simulink library "Storage_Type_5"  (R2018b)
settings: Solver=ode45  StartTime=0.0  StopTime=10.0  RelTol=1e-3  EnableMultiTasking=on
undefined symbols (not defined in the file): path_carnot
libraries: carnot x12
settings Model: Creator=bernd.hafner  LastModifiedBy=drhf
settings DataIOCC: LimitDataPoints=on  SaveFormat=Array  SignalLoggingSaveFormat=ModelDataLogs
settings OptimizationCC: ExpressionDepthLimit=2147483647  LifeSpan=inf
settings DebuggingCC: UnderspecifiedInitializationDetection=Classic  MergeDetectMultiDrivingBlocksExec=none  SolverPrmCheckMsg=warning  FcnCallInpInsideContextMsg=warning  StateNameClashWarn=warning  SFUnexpectedBacktrackingDiag=warning  SFNoUnconditionalDefaultTransitionDiag=warning  SFExecutionAtInitializationDiag=none
settings HardwareCC: ProdBitPerPointer=32  ProdBitPerSizeT=32  ProdBitPerPtrDiffT=32  ProdLargestAtomicFloat=None  ProdIntDivRoundTo=Undefined  ProdEndianess=Unspecified  ProdWordSize=32  ProdHWDeviceType=32-bit Generic
settings ModelReferenceCC: PropagateSignalLabelsOutOfModel=off
settings SFSimCC: SimUseLocalCustomCode=off
settings RTWCC: RTWUseLocalCustomCode=off
settings CodeAppCC: StateflowObjectComments=on
settings GRTTargetCC: TargetLangStandard=C89/C90 (ANSI)  CombineOutputUpdateFcns=off  GRTInterface=on
settings ConfigComp: CovMetricSettings=dw  CovHtmlReporting=on  CovSaveCumulativeToWorkspaceVar=on  CovSaveSingleToWorkspaceVar=on  CovExternalEMLEnable=off

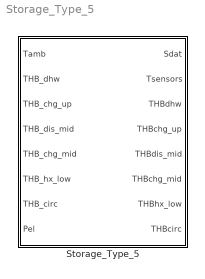
== system Storage_Type_5 ==
  Storage_Type_5 : Subsystem  mask(Combi-storage for hot water production and heating){t0=[10:5:55], hgt=1.7623, stgtype=5, tini=[10 12.3684210526316 14.7368421052632 17.1052631578947 19.4736842105263 21.8421052631579 24.2105263157895 26.5789473684211 28.9473684210526 31.3157894736842 33.6842105263158 36.0526315789474 38.4210526315789 40.7894736842105 43.1578947368421 45.5263157894737 47.8947368421053 50.2631578947368 52.6315789473684 55], mpts=[1 3 5 7 9 11 13 15 17 19], PathName=fullfile(path_carnot('libsl'), 'Storage', 'Thermal', 'Storage_Type_5', 'parameter_set'), FileName='StorageType5_800_L.mat', userPath=off, userParam=off, uwall=1, ubot=1, utop=1, axcond=1, volume=1, dia=0.85, standing=standing cylinder, nodes=20, mpoints=10, Tsensor=[0.2 0.5 0.7], pipe3inlet=1, pipe3outlet=0.6, pipe3dia=0.05, pipe1inlet=0.55, pipe1outlet=0.45, pipe1dia=0.05, hx1inlet=0.4, hx1outlet=0, hx1dia=0.03, hx1uac=200, hx1uam=0.15, hx1uat=0.6, hx1_uat2=0, hx1dplin=20, hx1dpqua=20, pipe2inlet=0.45, pipe2outlet=0.55, pipe2dia=0.05, hx2inlet=0, hx2outlet=1, hx2dia=0.025, hx2uac=450, hx2uam=0.4, hx2uat=0.8, hx2_uat2=0, hx2dplin=200, hx2dpqua=200, hx3inlet=0.9, hx3outlet=1, hx3dia=0.01, hx3uac=100, hx3uam=0, hx3uat=0, hx3_uat2=0, hx3dplin=10, hx3dpqua=10, heater1start=0.6, heater1end=0.65}
      mask prompts: t0 "Initial temperature (vector or scalar) in °C"; hgt "Height of storage in m"; stgtype "Storage Type (0..5)"; tini "Start temperatures of nodes in °C"; mpts "Index to measured nodes"; PathName "Path"; FileName "Parameter set"; userPath "Edit path and name of parameter set"; userParam "User defined parameters"; uwall "Heat transfer coefficient to ambient [W/m²K]"; ubot "Heat transfer coefficient to ambient bottom [W/m²K]"; utop "Heat transfer coefficient to ambient top [W/m²K]"; axcond "Effective thermal conductivity [W/m/K]"; volume "Volume [m³]"; dia "Diameter [m]"; standing "Position"; nodes "Number of nodes"; mpoints "Number of node temperatures (for display)"; Tsensor "Temperature sensor position (0..1, 0 = bottom, 1 = top)"; pipe3inlet "relative height of inlet, range from 0 (= bottom) to 1 (= top)"; pipe3outlet "relative height of outlet, range from 0 (= bottom) to 1 (= top)"; pipe3dia "Diameter of pipe in m"; pipe1inlet "relative height of inlet, range from 0 (= bottom) to 1 (= top)"; pipe1outlet "relative height of outlet, range from 0 (= bottom) to 1 (= top)"; pipe1dia "Diameter of pipe in m"; hx1inlet "relative height of inlet"; hx1outlet "relative height of outlet"; hx1dia "Diameter of HX pipe [m]"; hx1uac "uac: heat transfer coefficient [W/K /(kg/s) /(°C)]"; hx1uam "uam: massflow dependent heat transfer [-]"; hx1uat "uat: temperature dependent heat transfer [-]"; hx1_uat2 "uat2: temperature difference dependent heat transfer [-]"; hx1dplin "pressure drop linear in mdot [Pa*s/kg]"; hx1dpqua "pressure drop quadratic in mdot [Pa*s²/kg²]"; pipe2inlet "relative height of inlet, range from 0 (= bottom) to 1 (= top)"; pipe2outlet "relative height of outlet, range from 0 (= bottom) to 1 (= top)"; pipe2dia "Diameter of pipe in m"; hx2inlet "relative height of inlet"; hx2outlet "relative height of outlet"; hx2dia "Diameter of HX pipe [m]"; hx2uac "uac: heat transfer coefficient [W/K /(kg/s) /(°C)]"; hx2uam "uam: massflow dependent heat transfer [-]"; hx2uat "uat: temperature dependent heat transfer [-]"; hx2_uat2 "uat2: temperature difference dependent heat transfer [-]"; hx2dplin "pressure drop linear in mdot [Pa*s/kg]"; hx2dpqua "pressure drop quadratic in mdot [Pa*s²/kg²]"; hx3inlet "relative height of inlet"; hx3outlet "relative height of outlet"; hx3dia "Diameter of HX pipe [m]"; hx3uac "uac: constant heat transfer coefficient [W/K]"; hx3uam "uam: massflow dependent heat transfer [W*s/(K*kg)]"; hx3uat "uat: temperature dependent heat transfer [W/K²]"; hx3_uat2 "uat2: temperature difference dependent heat transfer [-]"; hx3dplin "Pressure drop coefficient dplin [Pa/(kg/s)]"; hx3dpqua "Pressure drop coefficient dpqua [Pa/(kg/s)²]"; heater1start "relative height start heating zone"; heater1end "relative height end heating zone"
      mask help:
      | Combi-storage for hot water production and heating.  The backup heater for the heating circuit is working on the storage.
      | The storage model has the following components (with their typical position):
      | - one solar heat exchanger (lower part)
      | - one hot water heat exchanger (total height)
      | - one hot water circulation heat exchanger (top part)
      | - one pipe connection for the heating circuit (middle part)
      | - one pipe connection for the backup heater (middle part)
      | - one pipe connection to heat the storage for hot water production (upper part )
      mask init:
      | [ok, param] = CarnotCallbacks_StorageConf('SetParam',stgtype,gcbh,PathName,FileName);
      mask Help: web(fullfile(path_carnot('help'),'Storage_Type_N.html'),'-helpbrowser')
      mask TypeOptions hgt: HX_EN12977_1/hgt | HX_EN12977_2/hgt | HX_EN12977_3/hgt | Pipe_Connection_1/hgt | Pipe_Connection_2/hgt | Pipe_Connection_3/hgt
      mask TypeOptions stgtype: CreateSdat/stgtype
      mask TypeOptions tini: sfun_storageTnodes/tini
      mask TypeOptions mpts: select_T/Indices
      mask Callback userPath: [ok, param] = CarnotCallbacks_StorageConf('UserEdit',5,gcbh);
      mask Callback userParam: [ok, param] = CarnotCallbacks_StorageConf('UserEdit',5,gcbh);
      mask TypeOptions uwall: sfun_storageTnodes/uloss
      mask TypeOptions ubot: sfun_storageTnodes/ubot
      mask TypeOptions utop: sfun_storageTnodes/utop
      mask TypeOptions axcond: sfun_storageTnodes/cond
      mask TypeOptions volume: sfun_storageTnodes/volume | CreateSdat/volume
      mask TypeOptions dia: sfun_storageTnodes/dia | Pipe_Connection_1/dstg | Pipe_Connection_2/dstg | Pipe_Connection_3/dstg
      mask TypeOptions standing: sfun_storageTnodes/standing
      mask TypeOptions nodes: sfun_storageTnodes/nodes | select_T/InputPortWidth | HX_EN12977_1/nodes | HX_EN12977_2/nodes | HX_EN12977_3/nodes | Pipe_Connection_1/nodes | Pipe_Connection_2/nodes | Pipe_Connection_3/nodes
      mask TypeOptions Tsensor: T_Sensor_Surface/pos
      mask TypeOptions pipe3inlet: Pipe_Connection_3/h_in
      mask TypeOptions pipe3outlet: Pipe_Connection_3/h_out
      mask TypeOptions pipe3dia: Pipe_Connection_3/dpipe
      mask TypeOptions pipe1inlet: Pipe_Connection_1/h_in
      mask TypeOptions pipe1outlet: Pipe_Connection_1/h_out
      mask TypeOptions pipe1dia: Pipe_Connection_1/dpipe
      mask TypeOptions hx1inlet: HX_EN12977_1/h_in
      mask TypeOptions hx1outlet: HX_EN12977_1/h_out
      mask TypeOptions hx1dia: HX_EN12977_1/dia
      mask TypeOptions hx1uac: HX_EN12977_1/ua0
      mask TypeOptions hx1uam: HX_EN12977_1/uam
      mask TypeOptions hx1uat: HX_EN12977_1/uat
      mask TypeOptions hx1_uat2: HX_EN12977_1/uat2
      mask TypeOptions hx1dplin: HX_EN12977_1/dplin
      mask TypeOptions hx1dpqua: HX_EN12977_1/dpqua
      mask TypeOptions pipe2inlet: Pipe_Connection_2/h_in
      mask TypeOptions pipe2outlet: Pipe_Connection_2/h_out
      mask TypeOptions pipe2dia: Pipe_Connection_2/dpipe
      mask TypeOptions hx2inlet: HX_EN12977_2/h_in
      mask TypeOptions hx2outlet: HX_EN12977_2/h_out
      mask TypeOptions hx2dia: HX_EN12977_2/dia
      mask TypeOptions hx2uac: HX_EN12977_2/ua0
      mask TypeOptions hx2uam: HX_EN12977_2/uam
      mask TypeOptions hx2uat: HX_EN12977_2/uat
      mask TypeOptions hx2_uat2: HX_EN12977_2/uat2
      mask TypeOptions hx2dplin: HX_EN12977_2/dplin
      mask TypeOptions hx2dpqua: HX_EN12977_2/dpqua
      mask TypeOptions hx3inlet: HX_EN12977_3/h_in
      mask TypeOptions hx3outlet: HX_EN12977_3/h_out
      mask TypeOptions hx3dia: HX_EN12977_3/dia
      mask TypeOptions hx3uac: HX_EN12977_3/ua0
      mask TypeOptions hx3uam: HX_EN12977_3/uam
      mask TypeOptions hx3uat: HX_EN12977_3/uat
      mask TypeOptions hx3_uat2: HX_EN12977_3/uat2
      mask TypeOptions hx3dplin: HX_EN12977_3/dplin
      mask TypeOptions hx3dpqua: HX_EN12977_3/dpqua
      mask TypeOptions heater1start: Electric_Heating_1/hin
      mask TypeOptions heater1end: Electric_Heating_1/hout
      mask DialogControl Container14 Prompt: Infos
      mask DialogControl ParameterGroupVar Prompt: Picking a parameter set
      mask DialogControl Control3 Prompt: Carnot public data
      mask DialogControl Control3 Callback: [ok, file] = CarnotCallbacks_StorageConf('GetFilename',5,gcbh,'public');
      mask DialogControl Control4 Prompt: Carnot internal data
      mask DialogControl Control4 Callback: [ok, file] = CarnotCallbacks_StorageConf('GetFilename',5,gcbh,'internal');
      mask DialogControl Control2 Prompt: Selected path
      mask DialogControl Control2 Callback: [ok, file] = CarnotCallbacks_StorageConf('GetFilename',5,gcbh,'selected');
      mask DialogControl Container4 Prompt: Parameter values
      mask DialogControl Container6 Prompt: Storage
      mask DialogControl Container8 Prompt: Connections
      mask DialogControl Container9 Prompt: Charging pipe (upper part)
      mask DialogControl Container10 Prompt: Charging pipe (middle part)
      mask DialogControl Container11 Prompt: Charging HX (lower part)
      mask DialogControl Container12 Prompt: Discharging pipe (house heating)
      mask DialogControl Container13 Prompt: HX DHW
      mask DialogControl Container16 Prompt: HX DHW circulation
      mask DialogControl Container17 Prompt: Electric Heating
      mask DialogControl Container18 Prompt: Heater 1
      mask DialogControl Control6 Prompt: Save in Carnot internal data
      mask DialogControl Control6 Callback: [ok, param] = CarnotCallbacks_StorageConf('SaveFilename',5,gcbh,'internal','STG');
      mask DialogControl Control5 Prompt: Save in selected path
      mask DialogControl Control5 Callback: [ok, param] = CarnotCallbacks_StorageConf('SaveFilename',5,gcbh,'selected','STG');
      mask Display:
      | % user defined picture file
      | namestr = ['Storage_Type_', num2str(get_param(gcb,'stgtype'))];
      | picfile = fullfile(path_carnot('intlibsl'), 'Storage','Thermal', ...
      |     namestr,'parameter_set', [namestr, '.jpg']);
      | 
      | % show internal picture if defined
      | pic = false;
      | if  ~BlockIsInCarnotLibrary       % if not located in library
      |     if exist(picfile, 'file')
      |         image(imread(picfile), [0.3, 0, 0.45, 1])
      |         set_param(gcb, 'BackgroundColor', 'White')
      |         pic = true;
      |     end
      | end
      | 
      | % show public picture
      | if ~pic
      |     set_param(gcb, 'BackgroundColor', 'Red')
      |     plot([36,36,40,50,54,54,50,40,36]/100,[90,50,45,45,50,90,93,93,90]/100, ...
      |         [36,51,40,51,36]/100,[50,50,68,85,85]/100,[36,51,44,51,36]/100, ...
      |         [54,54,56,58,58]/100,...
      |         [36,50,50,36]/100,[75,75,74,74]/100,...
      |         [36,34,34,36]/100,[75.5,75.5,73,73]/100)
      | end

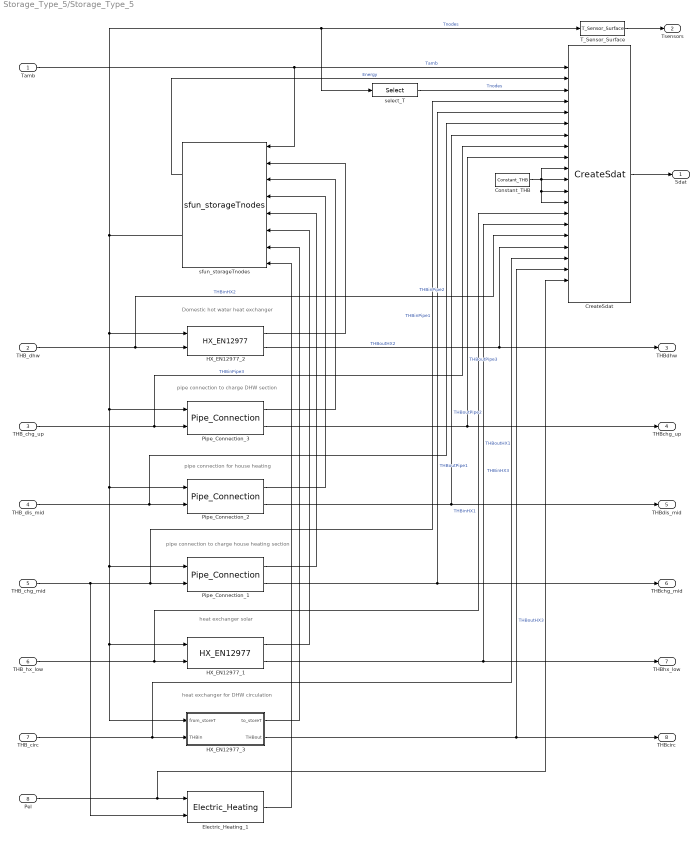
== system Storage_Type_5/Storage_Type_5 ==
  note: heat exchanger for DHW circulation
  note: heat exchanger solar
  note: pipe connection to charge house heating section
  note: pipe connection for house heating
  note: pipe connection to charge DHW section
  note: Domestic hot water heat exchanger
  Tamb : Inport
  THB_dhw : Inport  Port=2
  THB_chg_up : Inport  Port=3
  THB_dis_mid : Inport  Port=4
  THB_chg_mid : Inport  Port=5
  THB_hx_low : Inport  Port=6
  THB_circ : Inport  Port=7
  Pel : Inport  Port=8
  Constant_THB : carnot/Source/Simple/Constant_THB  t=20  mdot=0  p=1e5  mID=No Pressure Drop  fluid=Water  mix=0  mix2=0  mix3=0  dia=0.02  hgt=0
      settings: SourceProductName=Carnot
  CreateSdat : carnot/Basic/Thermal_Models/CreateSdat  volume=volume  stgtype=stgtype
      settings: SourceProductName=Carnot
  Electric_Heating_1 : carnot/Storage/Thermal/Storage_Ports/Electric_Heating  hin=heater1start  hout=heater1end  nodes=nodes
      settings: SourceProductName=Carnot
  HX_EN12977_1 : carnot/Storage/Thermal/Storage_Ports/HX_EN12977  h_in=hx1inlet  h_out=hx1outlet  hgt=hgt  dia=hx1dia  height=-0.70492  ua0=hx1uac  uam=hx1uam  uat=hx1uat  uat2=hx1_uat2  dplin=hx1dplin  dpqua=hx1dpqua  nodes=nodes
      settings: SourceProductName=Carnot
  HX_EN12977_2 : carnot/Storage/Thermal/Storage_Ports/HX_EN12977  h_in=hx2inlet  h_out=hx2outlet  hgt=hgt  dia=hx2dia  height=1.7623  ua0=hx2uac  uam=hx2uam  uat=hx2uat  uat2=hx2_uat2  dplin=hx2dplin  dpqua=hx2dpqua  nodes=nodes
      settings: SourceProductName=Carnot
  HX_EN12977_3 : Subsystem  mask(heat exchanger for storage, data EN 12977){h_in=hx3inlet, h_out=hx3outlet, hgt=hgt, dia=hx3dia, height=0.17623, ua0=hx3uac, uam=hx3uam, uat=hx3uat, uat2=hx3_uat2, dplin=hx3dplin, dpqua=hx3dpqua, nodes=nodes}
      mask prompts: h_in "relative height of inlet"; h_out "relative height of outlet"; hgt "Height of storage in m"; dia "Diameter of HX pipe [m]"; height "Height difference inlet-outlet [m]"; ua0 "uac: heat transfer coefficient [W/K /(kg/s) /(°C)]"; uam "uam: massflow dependent heat transfer [-]"; uat "uat: temperature dependent heat transfer [-]"; uat2 "uat2: temperature difference dependent heat transfer [-]"; dplin "Pressure drop coefficient dplin [Pa/(kg/s)]"; dpqua "Pressure drop coefficient dpqua [Pa/(kg/s)²]"; nodes "number of nodes"
      mask help:
      | The block transforms the incoming THV vector to a vector which the storage interprets as a heat exchanger.
      | Give inlet and outlet as a relative position 0=bottom to 1=top
      | The heat transfer is calculated by:
      | UA = uac * mdot^uam *
      |           ((Theatexchanger+Tstorage)/2)^uat *
      |           (Theatexchanger-Tstorage)^uat2
      mask init:
      | in = zeros(nodes,1);    % vector of length nodes
      | up = in;                % vector of length nodes
      | down = in;              % vector of length nodes
      | 
      | h_in = max(0,h_in);     % no nodes below 0
      | h_out = max(0,h_out);   % no nodes below 0
      | 
      | inlet = round(h_in*(nodes-1))+1;    % inlet position
      | outlet = round(h_out*(nodes-1))+1;  % outlet position
      | set_param(gcb,'height',num2str((h_out-h_in)*hgt));
      | % hgt = (h_out-h_in)*hgt;
      | 
      | in(inlet)=1;
      | 
      | if (h_in < h_out)           % if inlet below outlet
      |     up(inlet:outlet)=1;     % upwards
      | elseif (h_in > h_out)       % else if inlet above outlet
      |     down(outlet:inlet)=1;   % downwards
      | end
      mask Help: web(['file:///' fullfile(path_carnot('help'),'StoragePorts_HeatExchangerModels.html')],'-helpbrowser')
      mask TypeOptions dia: Pressure_Drop_StorageHX/dia
      mask TypeOptions height: Pressure_Drop_StorageHX/hgt
      mask TypeOptions ua0: sfun_storage_heatexchanger/p1
      mask TypeOptions uam: sfun_storage_heatexchanger/p2
      mask TypeOptions uat: sfun_storage_heatexchanger/p3
      mask TypeOptions uat2: sfun_storage_heatexchanger/p4
      mask TypeOptions dplin: Pressure_Drop_StorageHX/dplin
      mask TypeOptions dpqua: Pressure_Drop_StorageHX/dpqua
      mask TypeOptions nodes: sfun_storage_heatexchanger/nodes
      mask DialogControl ParameterTabVar0 Prompt: Geometry
      mask DialogControl ParameterTabVar01 Prompt: Heat transfer
      mask DialogControl ParameterTabVar012 Prompt: Pressure drop
      mask DialogControl ParameterTabVar0123 Prompt: Calculation
      mask Display: disp('HX EN12977')
  Pipe_Connection_1 : carnot/Storage/Thermal/Storage_Ports/Pipe_Connection  h_in=pipe1inlet  h_out=pipe1outlet  hgt=hgt  dpipe=pipe1dia  dstg=dia  height=-0.17623  nodes=nodes
      settings: SourceProductName=Carnot
  Pipe_Connection_2 : carnot/Storage/Thermal/Storage_Ports/Pipe_Connection  h_in=pipe2inlet  h_out=pipe2outlet  hgt=hgt  dpipe=pipe2dia  dstg=dia  height=0.17623  nodes=nodes
      settings: SourceProductName=Carnot
  Pipe_Connection_3 : carnot/Storage/Thermal/Storage_Ports/Pipe_Connection  h_in=pipe3inlet  h_out=pipe3outlet  hgt=hgt  dpipe=pipe3dia  dstg=dia  height=-0.70492  nodes=nodes
      settings: SourceProductName=Carnot
  T_Sensor_Surface : carnot/Control/T_Sensor_Surface  pos=Tsensor  tdel=10  t0=mean(tini)
      settings: SourceProductName=Carnot
  select_T : Selector  InputPortWidth=nodes  IndexOptions=Index vector (dialog)  Indices=[1 3 5 7 9 11 13 15 17 19]  OutputSizes=1
  sfun_storageTnodes : carnot/Basic/Thermal_Models/sfun_storageTnodes  uloss=uwall  ubot=ubot  utop=utop  cond=axcond  volume=volume  dia=dia  standing=standing cylinder  tini=tini  nodes=nodes  nconnect=7  elimthermocline=2  condinvtc=1e5
      settings: SourceProductName=Carnot
  Sdat : Outport
  Tsensors : Outport  Port=2
  THBdhw : Outport  Port=3
  THBchg_up : Outport  Port=4
  THBdis_mid : Outport  Port=5
  THBchg_mid : Outport  Port=6
  THBhx_low : Outport  Port=7
  THBcirc : Outport  Port=8
  wires:
  Constant_THB/1 -> CreateSdat/11, CreateSdat/13, CreateSdat/12, CreateSdat/10
  sfun_storageTnodes/1 -> CreateSdat/2  "Energy"
  Pipe_Connection_1/2 -> CreateSdat/5, THBchg_mid/1  "THBoutPipe1"
  Pipe_Connection_1/1 -> sfun_storageTnodes/5
  THB_chg_mid/1 -> Electric_Heating_1/2, Pipe_Connection_1/2, CreateSdat/4  "THBinPipe1"
  HX_EN12977_1/1 -> sfun_storageTnodes/6
  Pipe_Connection_2/2 -> CreateSdat/7, THBdis_mid/1  "THBoutPipe2"
  Pipe_Connection_2/1 -> sfun_storageTnodes/4
  THB_dis_mid/1 -> CreateSdat/6, Pipe_Connection_2/2  "THBinPipe2"
  Tamb/1 -> CreateSdat/1, sfun_storageTnodes/1  "Tamb"
  THB_dhw/1 -> HX_EN12977_2/2, CreateSdat/16  "THBinHX2"
  HX_EN12977_2/2 -> THBdhw/1, CreateSdat/17  "THBoutHX2"
  HX_EN12977_2/1 -> sfun_storageTnodes/2
  select_T/1 -> CreateSdat/3  "Tnodes"
  sfun_storageTnodes/2 -> Pipe_Connection_2/1, HX_EN12977_1/1, HX_EN12977_3/1(from_storeT), Pipe_Connection_1/1, Pipe_Connection_3/1, HX_EN12977_2/1, select_T/1, T_Sensor_Surface/1  "Tnodes"
  CreateSdat/1 -> Sdat/1
  THB_chg_up/1 -> Pipe_Connection_3/2, CreateSdat/8  "THBinPipe3"
  Pipe_Connection_3/2 -> CreateSdat/9, THBchg_up/1  "THBoutPipe3"
  Pipe_Connection_3/1 -> sfun_storageTnodes/3
  THB_hx_low/1 -> HX_EN12977_1/2, CreateSdat/14  "THBinHX1"
  HX_EN12977_1/2 -> THBhx_low/1, CreateSdat/15  "THBoutHX1"
  T_Sensor_Surface/1 -> Tsensors/1
  THB_circ/1 -> HX_EN12977_3/2(THBin), CreateSdat/18  "THBinHX3"
  HX_EN12977_3/1(to_storeT) -> sfun_storageTnodes/7
  HX_EN12977_3/2(THBout) -> THBcirc/1, CreateSdat/19  "THBoutHX3"
  Pel/1 -> Electric_Heating_1/1, CreateSdat/20
  Electric_Heating_1/1 -> sfun_storageTnodes/8

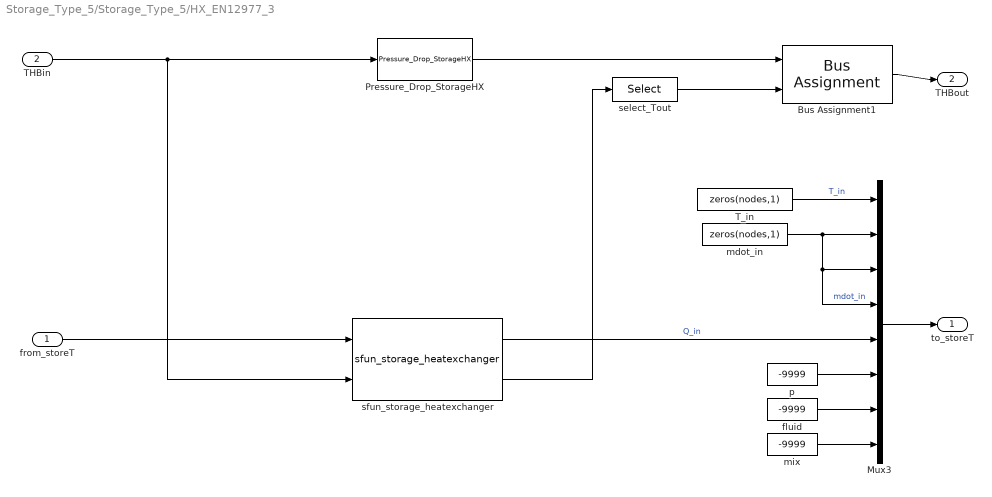
== system Storage_Type_5/Storage_Type_5/HX_EN12977_3 ==
  from_storeT : Inport
  THBin : Inport  Port=2
  Bus Assignment1 : BusAssignment  AssignedSignals=Temperature
  Mux3 : Mux  Inputs=8
  Pressure_Drop_StorageHX : carnot/Basic/Pressure_Drop/Pressure_Drop_StorageHX  dia=dia  hgt=height  dplin=dplin  dpqua=dpqua
      settings: SourceProductName=Carnot
  T_in : Constant  Value=zeros(nodes,1)
  fluid : Constant  Value=-9999
  mdot_in : Constant  Value=zeros(nodes,1)
  mix : Constant  Value=-9999
  p : Constant  Value=-9999
  select_Tout : Selector  InputPortWidth=nodes  IndexOptions=Index vector (dialog)  Indices=[outlet]  OutputSizes=1
  sfun_storage_heatexchanger : carnot/Basic/Thermal_Models/sfun_storage_heatexchanger  idn=heat transfer data fit EN12977  nodes=nodes  inlet=inlet  outlet=outlet  p1=ua0  p2=uam  p3=uat  p4=uat2  p5=0  p6=0  p7=0
      settings: SourceProductName=Carnot
  to_storeT : Outport
  THBout : Outport  Port=2
  wires:
  Pressure_Drop_StorageHX/1 -> Bus Assignment1/1
  sfun_storage_heatexchanger/2 -> select_Tout/1
  mix/1 -> Mux3/8
  fluid/1 -> Mux3/7
  p/1 -> Mux3/6
  Bus Assignment1/1 -> THBout/1
  sfun_storage_heatexchanger/1 -> Mux3/5  "Q_in"
  T_in/1 -> Mux3/1  "T_in"
  select_Tout/1 -> Bus Assignment1/2
  Mux3/1 -> to_storeT/1
  mdot_in/1 -> Mux3/4, Mux3/3, Mux3/2  "mdot_in"
  THBin/1 -> sfun_storage_heatexchanger/2, Pressure_Drop_StorageHX/1
  from_storeT/1 -> sfun_storage_heatexchanger/1
